simulink model "CoolingCheese_3rdPoint"  (R2022a)
settings: Solver=VariableStepAuto  StartTime=0.0  StopTime=H  RelTol=1e-3
undefined symbols (not defined in the file): C_c, C_f, k_af, k_fc, theta0_c, theta0_f, Ts, var_wc, var_wf
settings Model: Creator=mrnel  LastModifiedBy=mrnel

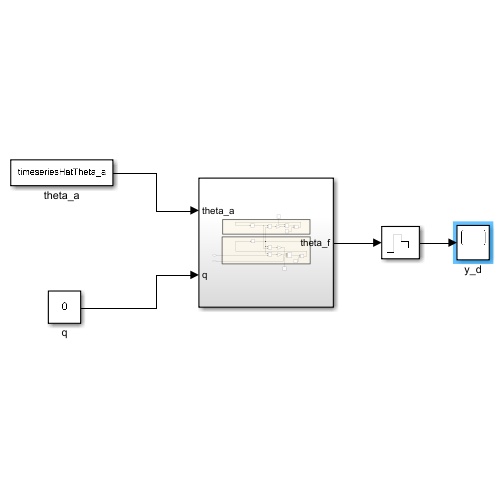
[thumbnail: Simulink's stored preview of the top-level diagram]
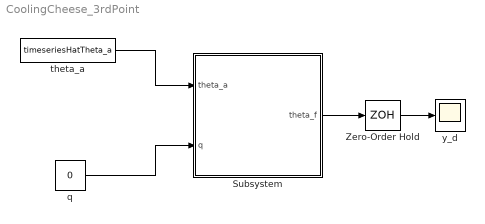
== system CoolingCheese_3rdPoint ==
  Subsystem : Subsystem
  Zero-Order Hold : ZeroOrderHold  SampleTime=Ts
  q : Constant  Value=0
  theta_a : FromWorkspace  VariableName=timeseriesHatTheta_a  SampleTime=Ts
  y_d : Scope
  wires:
  theta_a/1 -> Subsystem/1(theta_a)
  q/1 -> Subsystem/2(q)
  Subsystem/1(theta_f) -> Zero-Order Hold/1
  Zero-Order Hold/1 -> y_d/1

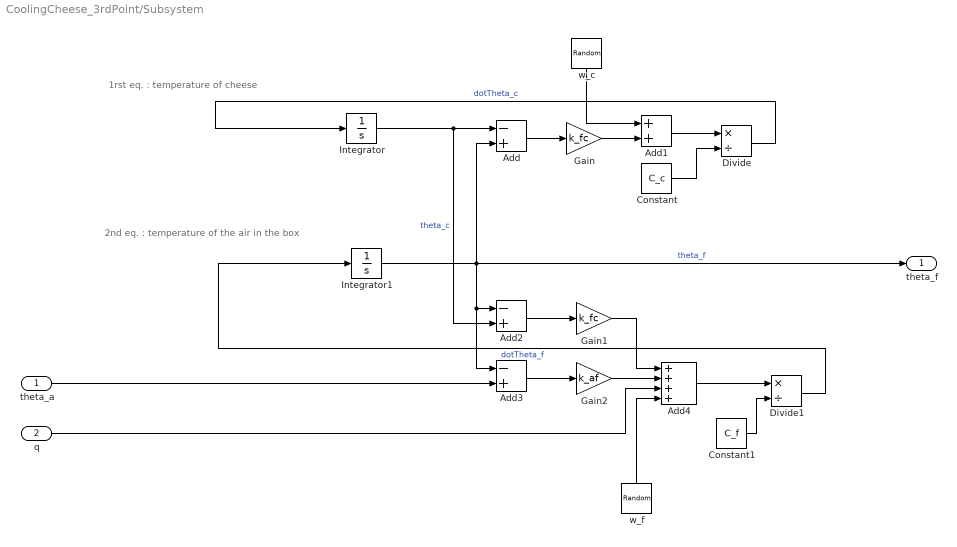
== system CoolingCheese_3rdPoint/Subsystem ==
  note: 2nd eq. : temperature of the air in the box
  note: 1rst eq. : temperature of cheese
  theta_a : Inport
  q : Inport  Port=2
  Add : Sum  Inputs=-+
  Add1 : Sum
  Add2 : Sum  Inputs=-+
  Add3 : Sum  Inputs=-+
  Add4 : Sum  Inputs=++++
  Constant : Constant  Value=C_c
  Constant1 : Constant  Value=C_f
  Divide : Product  Inputs=*/
  Divide1 : Product  Inputs=*/
  Gain : Gain  Gain=k_fc
  Gain1 : Gain  Gain=k_fc
  Gain2 : Gain  Gain=k_af
  Integrator : Integrator  InitialCondition=theta0_c
  Integrator1 : Integrator  InitialCondition=theta0_f
  w_c : RandomNumber  Variance=var_wc  SampleTime=Ts
  w_f : RandomNumber  Variance=var_wf  SampleTime=Ts
  theta_f : Outport
  wires:
  Gain2/1 -> Add4/2
  Divide/1 -> Integrator/1  "dotTheta_c"
  Add2/1 -> Gain1/1
  Add1/1 -> Divide/1
  Divide1/1 -> Integrator1/1  "dotTheta_f"
  w_c/1 -> Add1/1
  Integrator/1 -> Add2/2, Add/1  "theta_c"
  Integrator1/1 -> theta_f/1, Add3/1, Add2/1, Add/2  "theta_f"
  Gain/1 -> Add1/2
  Add/1 -> Gain/1
  Constant1/1 -> Divide1/2
  w_f/1 -> Add4/4
  Constant/1 -> Divide/2
  Gain1/1 -> Add4/1
  Add3/1 -> Gain2/1
  Add4/1 -> Divide1/1
  q/1 -> Add4/3
  theta_a/1 -> Add3/2
